simulink model "rob_zadanie2_sim2"  (R2023b)
settings: Solver=VariableStepAuto  StartTime=0.0  StopTime=50  RelTol=1e-3
undefined symbols (not defined in the file or in its folder): B1, B2, D1, D2, g, I1, I2, l1, l2, m1, m2, Mr, N1, N2, P1, P2, sp1, sp2, v12
libraries: slpidlib x2, SignalEditorBlockLib x1
settings Model: Creator=Filip  LastModifiedBy=Filip
settings DebuggingCC: AlgebraicLoopMsg=none

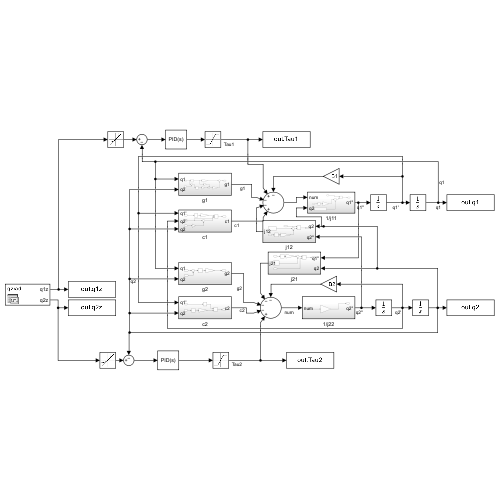
[thumbnail: Simulink's stored preview of the top-level diagram]
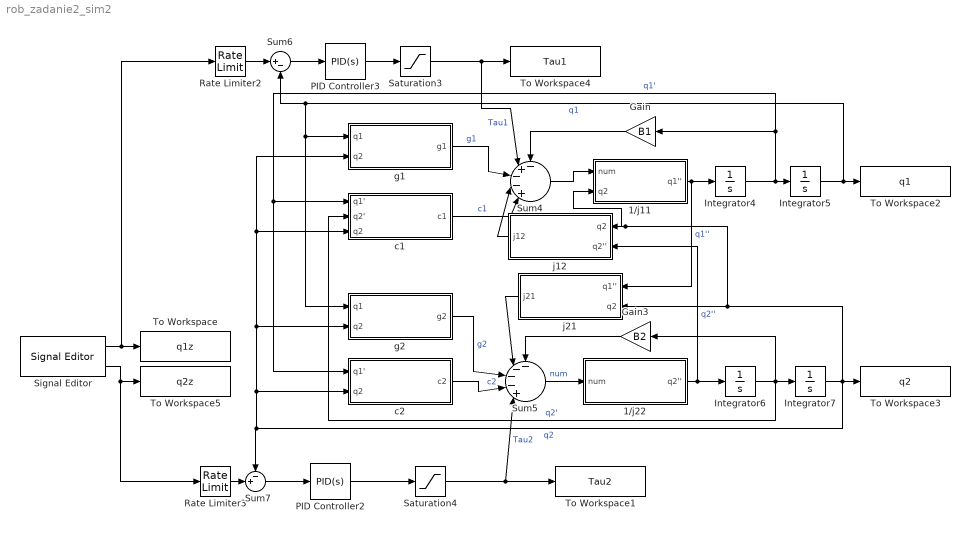
== system rob_zadanie2_sim2 ==
  1/j11 : Subsystem
  1/j22 : Subsystem
  Gain : Gain  Gain=B1
  Gain3 : Gain  Gain=B2
  Integrator4 : Integrator
  Integrator5 : Integrator  InitialCondition=sp1
  Integrator6 : Integrator
  Integrator7 : Integrator  InitialCondition=sp2
  PID Controller2 : slpidlib/PID Controller  Controller=PID  Form=Parallel  TimeDomain=Continuous-time  UseExternalTs=off  SampleTime=-1  IntegratorMethod=Forward Euler  FilterMethod=Forward Euler  ControllerParametersSource=internal  P=P2  I=I2  UseKiTs=off  D=D2  N=N2  UseFilter=on  TunerSelectOption=Transfer Function Based (PID Tuner App)  InitialConditionSource=internal  InitialConditionForIntegrator=0  InitialConditionForFilter=0  DifferentiatorICPrevScaledInput=0  ExternalReset=none  TrackingMode=off  Kt=1  LimitOutput=off  SatLimitsSource=internal  UpperSaturationLimit=inf  LowerSaturationLimit=-inf  LinearizeAsGain=on  AntiWindupMode=none  Kb=1  LimitIntegrator=off  UpperIntegratorSaturationLimit=inf  LowerIntegratorSaturationLimit=-inf  POutMin=[]  POutMax=[]  IOutMin=[]  IOutMax=[]  DOutMin=[]  DOutMax=[]  NOutMin=[]  NOutMax=[]  SumOutMin=[]  SumOutMax=[]  SaturationOutMin=[]  SaturationOutMax=[]  PParamMin=[]  PParamMax=[]  IParamMin=[]  IParamMax=[]  DParamMin=[]  DParamMax=[]  NParamMin=[]  NParamMax=[]  KbParamMin=[]  KbParamMax=[]  KtParamMin=[]  KtParamMax=[]  KbOutMin=[]  KbOutMax=[]  KtOutMin=[]  KtOutMax=[]  IntegratorOutMin=[]  IntegratorOutMax=[]  FilterOutMin=[]  FilterOutMax=[]  SumI1OutMin=[]  SumI1OutMax=[]  SumI2OutMin=[]  SumI2OutMax=[]  SumI3OutMin=[]  SumI3OutMax=[]  SumI4OutMin=[]  SumI4OutMax=[]  SumDOutMin=[]  SumDOutMax=[]  DifferentiatorOutMin=[]  DifferentiatorOutMax=[]  FilterDiffOutCoefMin=[]  FilterDiffOutCoefMax=[]  ReciprocalOutMin=[]  ReciprocalOutMax=[]  SumDenOutMin=[]  SumDenOutMax=[]  SumNumOutMin=[]  SumNumOutMax=[]  DivideOutMin=[]  DivideOutMax=[]  UdiffTsProdOutMin=[]  UdiffTsProdOutMax=[]  NTsProdOutMin=[]  NTsProdOutMax=[]  UintegralTsProdOutMin=[]  UintegralTsProdOutMax=[]  UngainTsProdOutMin=[]  UngainTsProdOutMax=[]  ClampingZeroOutDataTypeStr=Inherit: Inherit via back propagation  ClampingZeroOutMin=[]  ClampingZeroOutMax=[]  FilterDenConstantOutDataTypeStr=Inherit: Inherit via back propagation  FilterDenConstantOutMin=[]  FilterDenConstantOutMax=[]  PCopyOutDataTypeStr=Inherit: Inherit via back propagation  PCopyOutMin=[]  PCopyOutMax=[]  NCopyOutDataTypeStr=Inherit: Inherit via back propagation  NCopyOutMin=[]  NCopyOutMax=[]  IntegratorContinuousStateAttributes=''  IntegratorStateMustResolveToSignalObject=off  IntegratorRTWStateStorageClass=Auto  FilterContinuousStateAttributes=''  FilterStateMustResolveToSignalObject=off  FilterRTWStateStorageClass=Auto  ParallelPVariant=InternalParameters  IdealPVariant=Disabled  IVariant=InternalParameters  DVariant=InternalParameters  IntegratorVariant=Continuous  SatVariant=Disabled  AWVariant=Passthrough  PCopyVariant=Disabled  TRVariant=Disabled  FdbkBlocksVariant=Forward  IdealPFdbkVariant=Disabled  SatFdbkVariant=Disabled  DerivativeFilterVariant=ContFilter  NVariant=InternalParameters  NCopyVariant=Disabled  FilterICVariant=InternalICsFilter  IntegratorICVariant=InternalICs  ExternalResetVariant=Disabled  TRSumVariant=Passthrough  SumFdbkVariant=Disabled  SumVariant=Sum_PID  TsampFilterVariant=InternalTs  TsampNgainVariant=Passthrough  TsampIntegralVariant=Disabled_SignalSpec  ExternalSaturationOutDataTypeStr=Inherit: Same as second input
  PID Controller3 : slpidlib/PID Controller  Controller=PID  Form=Parallel  TimeDomain=Continuous-time  UseExternalTs=off  SampleTime=-1  IntegratorMethod=Forward Euler  FilterMethod=Forward Euler  ControllerParametersSource=internal  P=P1  I=I1  UseKiTs=off  D=D1  N=N1  UseFilter=on  TunerSelectOption=Transfer Function Based (PID Tuner App)  InitialConditionSource=internal  InitialConditionForIntegrator=0  InitialConditionForFilter=0  DifferentiatorICPrevScaledInput=0  ExternalReset=none  TrackingMode=off  Kt=1  LimitOutput=off  SatLimitsSource=internal  UpperSaturationLimit=inf  LowerSaturationLimit=-inf  LinearizeAsGain=on  AntiWindupMode=none  Kb=1  LimitIntegrator=off  UpperIntegratorSaturationLimit=inf  LowerIntegratorSaturationLimit=-inf  POutMin=[]  POutMax=[]  IOutMin=[]  IOutMax=[]  DOutMin=[]  DOutMax=[]  NOutMin=[]  NOutMax=[]  SumOutMin=[]  SumOutMax=[]  SaturationOutMin=[]  SaturationOutMax=[]  PParamMin=[]  PParamMax=[]  IParamMin=[]  IParamMax=[]  DParamMin=[]  DParamMax=[]  NParamMin=[]  NParamMax=[]  KbParamMin=[]  KbParamMax=[]  KtParamMin=[]  KtParamMax=[]  KbOutMin=[]  KbOutMax=[]  KtOutMin=[]  KtOutMax=[]  IntegratorOutMin=[]  IntegratorOutMax=[]  FilterOutMin=[]  FilterOutMax=[]  SumI1OutMin=[]  SumI1OutMax=[]  SumI2OutMin=[]  SumI2OutMax=[]  SumI3OutMin=[]  SumI3OutMax=[]  SumI4OutMin=[]  SumI4OutMax=[]  SumDOutMin=[]  SumDOutMax=[]  DifferentiatorOutMin=[]  DifferentiatorOutMax=[]  FilterDiffOutCoefMin=[]  FilterDiffOutCoefMax=[]  ReciprocalOutMin=[]  ReciprocalOutMax=[]  SumDenOutMin=[]  SumDenOutMax=[]  SumNumOutMin=[]  SumNumOutMax=[]  DivideOutMin=[]  DivideOutMax=[]  UdiffTsProdOutMin=[]  UdiffTsProdOutMax=[]  NTsProdOutMin=[]  NTsProdOutMax=[]  UintegralTsProdOutMin=[]  UintegralTsProdOutMax=[]  UngainTsProdOutMin=[]  UngainTsProdOutMax=[]  ClampingZeroOutDataTypeStr=Inherit: Inherit via back propagation  ClampingZeroOutMin=[]  ClampingZeroOutMax=[]  FilterDenConstantOutDataTypeStr=Inherit: Inherit via back propagation  FilterDenConstantOutMin=[]  FilterDenConstantOutMax=[]  PCopyOutDataTypeStr=Inherit: Inherit via back propagation  PCopyOutMin=[]  PCopyOutMax=[]  NCopyOutDataTypeStr=Inherit: Inherit via back propagation  NCopyOutMin=[]  NCopyOutMax=[]  IntegratorContinuousStateAttributes=''  IntegratorStateMustResolveToSignalObject=off  IntegratorRTWStateStorageClass=Auto  FilterContinuousStateAttributes=''  FilterStateMustResolveToSignalObject=off  FilterRTWStateStorageClass=Auto  ParallelPVariant=InternalParameters  IdealPVariant=Disabled  IVariant=InternalParameters  DVariant=InternalParameters  IntegratorVariant=Continuous  SatVariant=Disabled  AWVariant=Passthrough  PCopyVariant=Disabled  TRVariant=Disabled  FdbkBlocksVariant=Forward  IdealPFdbkVariant=Disabled  SatFdbkVariant=Disabled  DerivativeFilterVariant=ContFilter  NVariant=InternalParameters  NCopyVariant=Disabled  FilterICVariant=InternalICsFilter  IntegratorICVariant=InternalICs  ExternalResetVariant=Disabled  TRSumVariant=Passthrough  SumFdbkVariant=Disabled  SumVariant=Sum_PID  TsampFilterVariant=InternalTs  TsampNgainVariant=Passthrough  TsampIntegralVariant=Disabled_SignalSpec  ExternalSaturationOutDataTypeStr=Inherit: Same as second input
  Rate Limiter2 : RateLimiter  RisingSlewLimit=v12  FallingSlewLimit=-v12
  Rate Limiter3 : RateLimiter  RisingSlewLimit=v12  FallingSlewLimit=-v12
  Saturation3 : Saturate  UpperLimit=Mr  LowerLimit=-Mr
  Saturation4 : Saturate  UpperLimit=Mr  LowerLimit=-Mr
  Signal Editor : SignalEditorBlockLib/Signal Editor  FileName=qz.mat  ActiveScenario=qzrad  ActiveSignal=q1z  IsBus=off  OutputBusObjectStr=Bus: BusObject  SampleTime=0  Interpolate=off  ZeroCross=off  OutputAfterFinalValue=Setting to zero  Unit=inherit  PreserveSignalName=on  ApplySigPropsToAllScenarios=on  ApplySigPropsToAllSignals=off
  Sum4 : Sum  Inputs=-+--+|
  Sum5 : Sum  Inputs=----+|
  Sum6 : Sum  Inputs=|+-
  Sum7 : Sum  Inputs=-+|
  To Workspace : ToWorkspace  VariableName=q1z  SampleTime=-1
  To Workspace1 : ToWorkspace  VariableName=Tau2  SampleTime=-1
  To Workspace2 : ToWorkspace  VariableName=q1  SampleTime=-1
  To Workspace3 : ToWorkspace  VariableName=q2  SampleTime=-1
  To Workspace4 : ToWorkspace  VariableName=Tau1  SampleTime=-1
  To Workspace5 : ToWorkspace  VariableName=q2z  SampleTime=-1
  c1 : Subsystem
  c2 : Subsystem
  g1 : Subsystem
  g2 : Subsystem
  j12 : Subsystem
  j21 : Subsystem
  wires:
  Saturation4/1 -> To Workspace1/1, Sum5/5  "Tau2"
  Gain3/1 -> Sum5/1
  1/j11/1(q1'') -> j21/1(q1''), Integrator4/1  "q1''"
  Integrator7/1 -> To Workspace3/1, 1/j11/2(q2), j12/1(q2), j21/2(q2), g2/2(q2), g1/2(q2), c1/3(q2), c2/2(q2), Sum7/1  "q2"
  Rate Limiter3/1 -> Sum7/2
  Signal Editor/2 -> Rate Limiter3/1, To Workspace5/1
  Sum7/1 -> PID Controller2/1
  j21/1(j21) -> Sum5/2
  PID Controller3/1 -> Saturation3/1
  Signal Editor/1 -> Rate Limiter2/1, To Workspace/1
  PID Controller2/1 -> Saturation4/1
  Saturation3/1 -> To Workspace4/1, Sum4/2  "Tau1"
  g2/1(g2) -> Sum5/3  "g2"
  Integrator5/1 -> To Workspace2/1, Sum6/2, g2/1(q1), g1/1(q1)  "q1"
  Gain/1 -> Sum4/1
  Sum5/1 -> 1/j22/1(num)  "num"
  Integrator6/1 -> Gain3/1, c1/2(q2'), Integrator7/1  "q2'"
  Sum6/1 -> PID Controller3/1
  g1/1(g1) -> Sum4/3  "g1"
  1/j22/1(q2'') -> j12/2(q2''), Integrator6/1  "q2''"
  c2/1(c2) -> Sum5/4  "c2"
  Sum4/1 -> 1/j11/1(num)
  Integrator4/1 -> Integrator5/1, c2/1(q1'), c1/1(q1'), Gain/1  "q1'"
  j12/1(j12) -> Sum4/4
  c1/1(c1) -> Sum4/5  "c1"
  Rate Limiter2/1 -> Sum6/1

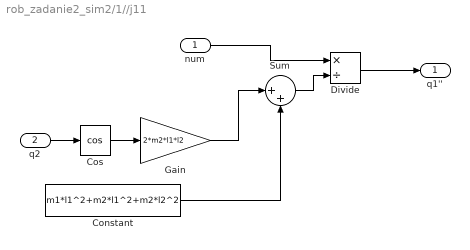
== system rob_zadanie2_sim2/1//j11 ==
  num : Inport
  q2 : Inport  Port=2
  Constant : Constant  Value=m1*l1^2+m2*l1^2+m2*l2^2
  Cos : Trigonometry  Operator=cos
  Divide : Product  Inputs=*/
  Gain : Gain  Gain=2*m2*l1*l2
  Sum : Sum  Inputs=|++
  q1'' : Outport
  wires:
  q2/1 -> Cos/1
  Cos/1 -> Gain/1
  Gain/1 -> Sum/1
  Constant/1 -> Sum/2
  num/1 -> Divide/1
  Sum/1 -> Divide/2
  Divide/1 -> q1''/1

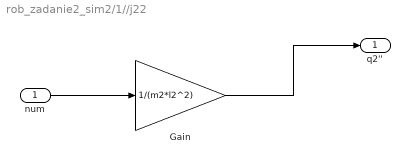
== system rob_zadanie2_sim2/1//j22 ==
  num : Inport
  Gain : Gain  Gain=1/(m2*l2^2)
  q2'' : Outport
  wires:
  num/1 -> Gain/1
  Gain/1 -> q2''/1

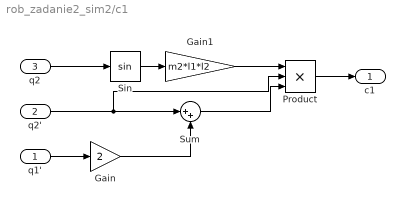
== system rob_zadanie2_sim2/c1 ==
  q1' : Inport
  q2' : Inport  Port=2
  q2 : Inport  Port=3
  Gain : Gain  Gain=2
  Gain1 : Gain  Gain=m2*l1*l2
  Product : Product  Inputs=3
  Sin : Trigonometry
  Sum : Sum  Inputs=|++
  c1 : Outport
  wires:
  q1'/1 -> Gain/1
  Gain/1 -> Sum/2
  q2'/1 -> Product/2, Sum/1
  q2/1 -> Sin/1
  Sin/1 -> Gain1/1
  Gain1/1 -> Product/1
  Product/1 -> c1/1
  Sum/1 -> Product/3

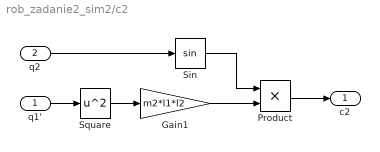
== system rob_zadanie2_sim2/c2 ==
  q1' : Inport
  q2 : Inport  Port=2
  Gain1 : Gain  Gain=m2*l1*l2
  Product : Product
  Sin : Trigonometry
  Square : Math  Operator=square
  c2 : Outport
  wires:
  q1'/1 -> Square/1
  Square/1 -> Gain1/1
  Gain1/1 -> Product/2
  q2/1 -> Sin/1
  Sin/1 -> Product/1
  Product/1 -> c2/1

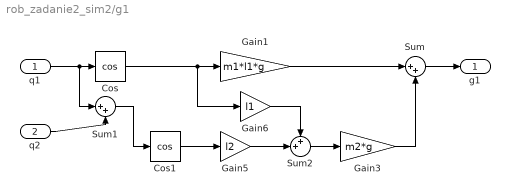
== system rob_zadanie2_sim2/g1 ==
  q1 : Inport
  q2 : Inport  Port=2
  Cos : Trigonometry  Operator=cos
  Cos1 : Trigonometry  Operator=cos
  Gain1 : Gain  Gain=m1*l1*g
  Gain3 : Gain  Gain=m2*g
  Gain5 : Gain  Gain=l2
  Gain6 : Gain  Gain=l1
  Sum : Sum  Inputs=|++
  Sum1 : Sum  Inputs=|++
  Sum2 : Sum  Inputs=++|
  g1 : Outport
  wires:
  q1/1 -> Sum1/1, Cos/1
  Cos/1 -> Gain1/1, Gain6/1
  q2/1 -> Sum1/2
  Sum1/1 -> Cos1/1
  Cos1/1 -> Gain5/1
  Gain5/1 -> Sum2/2
  Gain6/1 -> Sum2/1
  Sum2/1 -> Gain3/1
  Gain3/1 -> Sum/2
  Sum/1 -> g1/1
  Gain1/1 -> Sum/1

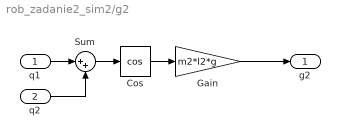
== system rob_zadanie2_sim2/g2 ==
  q1 : Inport
  q2 : Inport  Port=2
  Cos : Trigonometry  Operator=cos
  Gain : Gain  Gain=m2*l2*g
  Sum : Sum  Inputs=|++
  g2 : Outport
  wires:
  q1/1 -> Sum/1
  q2/1 -> Sum/2
  Sum/1 -> Cos/1
  Cos/1 -> Gain/1
  Gain/1 -> g2/1

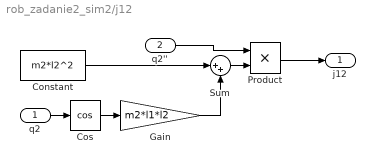
== system rob_zadanie2_sim2/j12 ==
  q2 : Inport
  q2'' : Inport  Port=2
  Constant : Constant  Value=m2*l2^2  SampleTime=-1
  Cos : Trigonometry  Operator=cos
  Gain : Gain  Gain=m2*l1*l2
  Product : Product
  Sum : Sum  Inputs=|++
  j12 : Outport
  wires:
  q2/1 -> Cos/1
  Cos/1 -> Gain/1
  Gain/1 -> Sum/2
  Constant/1 -> Sum/1
  Sum/1 -> Product/2
  q2''/1 -> Product/1
  Product/1 -> j12/1

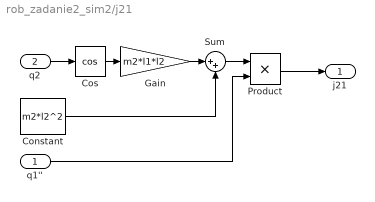
== system rob_zadanie2_sim2/j21 ==
  q1'' : Inport
  q2 : Inport  Port=2
  Constant : Constant  Value=m2*l2^2
  Cos : Trigonometry  Operator=cos
  Gain : Gain  Gain=m2*l1*l2
  Product : Product
  Sum : Sum  Inputs=|++
  j21 : Outport
  wires:
  q2/1 -> Cos/1
  Cos/1 -> Gain/1
  Gain/1 -> Sum/1
  Sum/1 -> Product/1
  q1''/1 -> Product/2
  Product/1 -> j21/1
  Constant/1 -> Sum/2
